simulink model "L1AdaptiveSystemModel"  (Simulink 7.3)
settings: Solver=ode45  StartTime=0.0  StopTime=30  RelTol=1e-3
InitFcn:
  | initL1AdaptiveSystemModel
StopFcn:
  | plotlab
values from neighbouring files (symbols this model uses):
  A = [0 1;0 0]    [initL1AdaptiveSystemModel.m]
  Am = A - b*km'    [initL1AdaptiveSystemModel.m]
  b = [0 ; d0]    [initL1AdaptiveSystemModel.m]
  c = [1 ; 1]    [initL1AdaptiveSystemModel.m]
  Cs_den = [1 25]    [initL1AdaptiveSystemModel.m]
  Cs_num = 25    [initL1AdaptiveSystemModel.m]
  Gamma = 100    [initL1AdaptiveSystemModel.m]
  kg = -(c'*(Am^-1)*b).^-1    [initL1AdaptiveSystemModel.m]
  km = [0.25 ; 0.707]    [initL1AdaptiveSystemModel.m]
  P = lyap(Am',Q)    [initL1AdaptiveSystemModel.m]
  theta = [0 -0.018 0.015 -0.062 0.0095 0.021]    [initL1AdaptiveSystemModel.m]
  theta2 = [4 -0.018 0.015 -0.062 0.0095 0.021]    [initL1AdaptiveSystemModel.m]
  ththat0 = zeros(6,1)    [initL1AdaptiveSystemModel.m]
  tNonlinChange = 10    [initL1AdaptiveSystemModel.m]
  tNonlinEnable = 0    [initL1AdaptiveSystemModel.m]
  x0 = zeros(2,1)    [initL1AdaptiveSystemModel.m]
  xhat0 = zeros(2,1)    [initL1AdaptiveSystemModel.m]
libraries: dspmtrx3 x4, simulink x3, Projection x1
settings Model: Creator=alp.marangoz  LastModifiedBy=Alp
settings OptimizationCC: ExpressionDepthLimit=128
settings DebuggingCC: StateNameClashWarn=none  StrictBusMsg=ErrorLevel1
settings CodeAppCC: CustomSymbolStrType=$N$R$M_T
settings GRTTargetCC: CombineOutputUpdateFcns=on

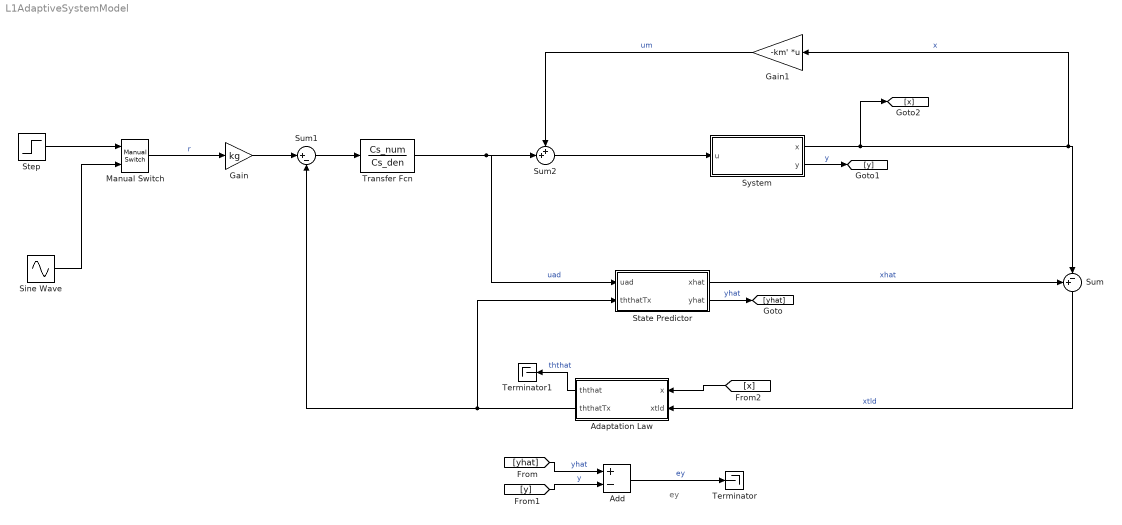
== system L1AdaptiveSystemModel ==
  note: ey
  Adaptation Law : Subsystem  TreatAsAtomicUnit=on
      settings: MinAlgLoopOccurrences=on
  Add : Sum  Inputs=+-  OutDataType=fixdt(1, 16)  OutScaling=2^-10
  Gain : Gain  Gain=kg  ParameterDataType=fixdt(1, 16)  ParameterScaling=2^0  OutDataType=fixdt(1, 16)  OutScaling=2^0
  Gain1 : Gain  Gain=-km'  Multiplication=Matrix(K*u)  ParameterDataType=fixdt(1, 16)  ParameterScaling=2^0  OutDataType=fixdt(1, 16)  OutScaling=2^0
  Manual Switch : simulink/Signal Routing/Manual Switch  SystemSampleTime=-1  sw=0  action=0  varsize=off
  Sine Wave : Sin  Amplitude=-2  Bias=0  Frequency=0.15  Phase=0  Samples=10  SampleTime=0  Offset=0
  State Predictor : Subsystem  TreatAsAtomicUnit=on
      settings: MinAlgLoopOccurrences=on
  Step : Step  SampleTime=0  VectorParams1D=off
  Sum : Sum  Inputs=+-|  OutDataType=fixdt(1, 16)  OutScaling=2^0
  Sum1 : Sum  Inputs=|+-  OutDataType=fixdt(1, 16)  OutScaling=2^0
  Sum2 : Sum  Inputs=++|  OutDataType=fixdt(1, 16)  OutScaling=2^0
  System : Subsystem  TreatAsAtomicUnit=on
      settings: MinAlgLoopOccurrences=on
  Terminator : Terminator
  Terminator1 : Terminator
  Transfer Fcn : TransferFcn  Numerator=Cs_num  Denominator=Cs_den
  wires:
  Sum/1 -> Adaptation Law/2(xtld)  "xtld"
  Manual Switch/1 -> Gain/1  "r"
  State Predictor/2(yhat) -> [yhat]  "yhat"
  System/2(y) -> [y]  "y"
  [yhat] -> Add/1  "yhat"
  [y] -> Add/2  "y"
  Add/1 -> Terminator/1  "ey"
  Step/1 -> Manual Switch/1
  Sine Wave/1 -> Manual Switch/2
  System/1(x) -> [x], Sum/2, Gain1/1  "x"
  Gain/1 -> Sum1/1
  State Predictor/1(xhat) -> Sum/1  "xhat"
  Sum1/1 -> Transfer Fcn/1
  Transfer Fcn/1 -> State Predictor/1(uad), Sum2/2  "uad"
  Adaptation Law/2(ththatTx) -> Sum1/2, State Predictor/2(ththatTx)
  Adaptation Law/1(ththat) -> Terminator1/1  "ththat"
  [x] -> Adaptation Law/1(x)
  Sum2/1 -> System/1(u)
  Gain1/1 -> Sum2/1  "um"

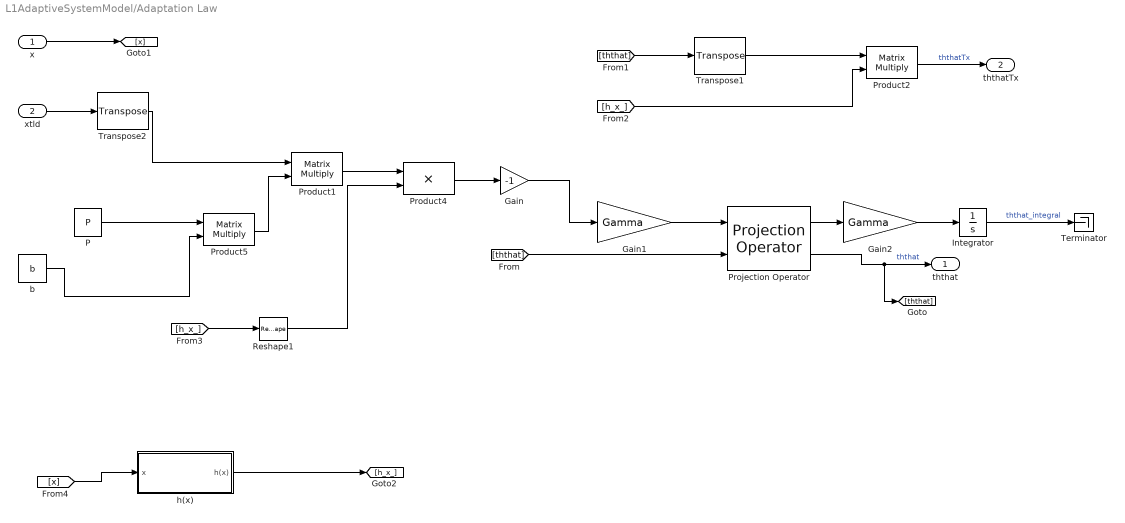
== system L1AdaptiveSystemModel/Adaptation Law ==
  x : Inport  OutDataType=fixdt(1, 16)  OutScaling=2^0
  xtld : Inport  Port=2  OutDataType=fixdt(1, 16)  OutScaling=2^0
  Gain : Gain  Gain=-1  ParameterDataType=fixdt(1, 16)  ParameterScaling=2^0  OutDataType=fixdt(1, 16)  OutScaling=2^0
  Gain1 : Gain  Gain=Gamma  ParameterDataType=fixdt(1, 16)  ParameterScaling=2^0  OutDataType=fixdt(1, 16)  OutScaling=2^0
  Gain2 : Gain  Gain=Gamma  ParameterDataType=fixdt(1, 16)  ParameterScaling=2^0  OutDataType=fixdt(1, 16)  OutScaling=2^0
  Integrator : Integrator  InitialCondition=ththat0
  P : Constant  Value=P  VectorParams1D=off  OutDataType=fixdt(1, 16)  OutScaling=2^0
  Product1 : Product  Multiplication=Matrix(*)  OutDataType=fixdt(1, 16)  OutScaling=2^0  RndMeth=Zero
  Product2 : Product  Multiplication=Matrix(*)  OutDataType=fixdt(1, 16)  OutScaling=2^0  RndMeth=Zero
  Product4 : Product  OutDataType=fixdt(1, 16)  OutScaling=2^0  RndMeth=Zero
  Product5 : Product  Multiplication=Matrix(*)  OutDataType=fixdt(1, 16)  OutScaling=2^0  RndMeth=Zero
  Projection Operator : Projection/Projection Operator  SystemSampleTime=-1  EpsilonTheta=.1  Prmax=1  Prcenter=0  Pr0=ththat0
  Reshape1 : Reshape  OutputDimensionality=Column vector (2-D)  OutputDimensions=[1]
  Terminator : Terminator
  Transpose1 : dspmtrx3/Transpose  SystemSampleTime=-1  Hermitian=off  overflowFlag=off
  Transpose2 : dspmtrx3/Transpose  SystemSampleTime=-1  Hermitian=off  overflowFlag=off
  b : Constant  Value=b  VectorParams1D=off  OutDataType=fixdt(1, 16)  OutScaling=2^0
  h(x) : Subsystem  TreatAsAtomicUnit=on
  ththat : Outport  OutDataType=fixdt(1, 16)  OutScaling=2^0
  ththatTx : Outport  Port=2  OutDataType=fixdt(1, 16)  OutScaling=2^0
  wires:
  P/1 -> Product5/1
  xtld/1 -> Transpose2/1
  Transpose2/1 -> Product1/1
  Product5/1 -> Product1/2
  b/1 -> Product5/2
  Gain/1 -> Gain1/1
  Gain1/1 -> Projection Operator/1
  Projection Operator/1 -> Gain2/1
  Gain2/1 -> Integrator/1
  Projection Operator/2 -> ththat/1, [ththat]  "ththat"
  Integrator/1 -> Terminator/1  "ththat_integral"
  Transpose1/1 -> Product2/1
  Product2/1 -> ththatTx/1  "ththatTx"
  [ththat] -> Transpose1/1
  [h_x_] -> Product2/2
  [ththat] -> Projection Operator/2
  x/1 -> [x]
  Product4/1 -> Gain/1
  [h_x_] -> Reshape1/1
  Reshape1/1 -> Product4/2
  Product1/1 -> Product4/1
  [x] -> h(x)/1(x)
  h(x)/1(h(x)) -> [h_x_]

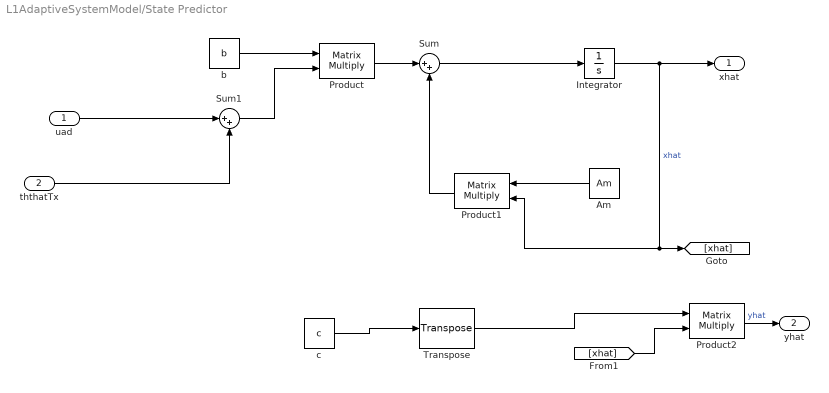
== system L1AdaptiveSystemModel/State Predictor ==
  uad : Inport  OutDataType=fixdt(1, 16)  OutScaling=2^0
  ththatTx : Inport  Port=2  OutDataType=fixdt(1, 16)  OutScaling=2^0
  Am : Constant  Value=Am  VectorParams1D=off  OutDataType=fixdt(1, 16)  OutScaling=2^0
  Integrator : Integrator  InitialCondition=xhat0
  Product : Product  Multiplication=Matrix(*)  OutDataType=fixdt(1, 16)  OutScaling=2^0  RndMeth=Zero
  Product1 : Product  Multiplication=Matrix(*)  OutDataType=fixdt(1, 16)  OutScaling=2^0  RndMeth=Zero
  Product2 : Product  Multiplication=Matrix(*)  OutDataType=fixdt(1, 16)  OutScaling=2^0  RndMeth=Zero
  Sum : Sum  Inputs=|++  OutDataType=fixdt(1, 16)  OutScaling=2^0
  Sum1 : Sum  Inputs=|++  OutDataType=fixdt(1, 16)  OutScaling=2^0
  Transpose : dspmtrx3/Transpose  SystemSampleTime=-1  Hermitian=off  overflowFlag=off
  b : Constant  Value=b  VectorParams1D=off  OutDataType=fixdt(1, 16)  OutScaling=2^0
  c : Constant  Value=c  VectorParams1D=off  OutDataType=fixdt(1, 16)  OutScaling=2^0
  xhat : Outport  OutDataType=fixdt(1, 16)  OutScaling=2^0
  yhat : Outport  Port=2  OutDataType=fixdt(1, 16)  OutScaling=2^0
  wires:
  c/1 -> Transpose/1
  Am/1 -> Product1/1
  Sum/1 -> Integrator/1
  Integrator/1 -> xhat/1, Product1/2, [xhat]  "xhat"
  Product1/1 -> Sum/2
  Product/1 -> Sum/1
  Transpose/1 -> Product2/1
  Product2/1 -> yhat/1  "yhat"
  b/1 -> Product/1
  Sum1/1 -> Product/2
  uad/1 -> Sum1/1
  [xhat] -> Product2/2
  ththatTx/1 -> Sum1/2

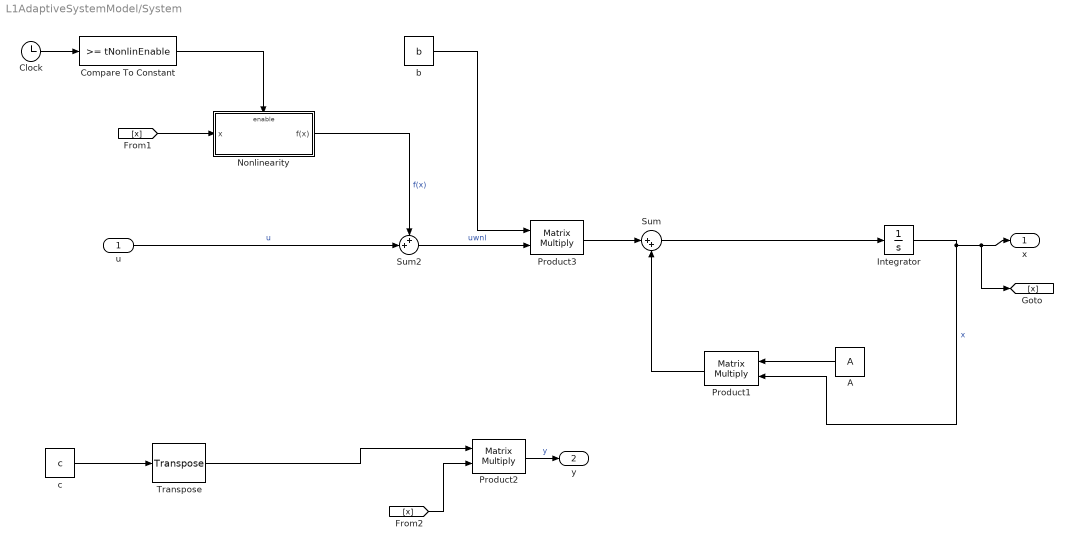
== system L1AdaptiveSystemModel/System ==
  u : Inport  OutDataType=fixdt(1, 16)  OutScaling=2^0
  A : Constant  Value=A  VectorParams1D=off  OutDataType=fixdt(1, 16)  OutScaling=2^0
  Clock : Clock
      settings: Decimation=10
  Compare To Constant : simulink/Logic and Bit Operations/Compare To Constant  SystemSampleTime=-1  relop=>=  const=tNonlinEnable  LogicOutDataTypeMode=uint8  ZeroCross=off
  Integrator : Integrator  InitialCondition=x0
  Nonlinearity : Subsystem  TreatAsAtomicUnit=on
  Product1 : Product  Multiplication=Matrix(*)  OutDataType=fixdt(1, 16)  OutScaling=2^0  RndMeth=Zero
  Product2 : Product  Multiplication=Matrix(*)  OutDataType=fixdt(1, 16)  OutScaling=2^0  RndMeth=Zero
  Product3 : Product  Multiplication=Matrix(*)  OutDataType=fixdt(1, 16)  OutScaling=2^0  RndMeth=Zero
  Sum : Sum  Inputs=|++  OutDataType=fixdt(1, 16)  OutScaling=2^0
  Sum2 : Sum  Inputs=++|  OutDataType=fixdt(1, 16)  OutScaling=2^0
  Transpose : dspmtrx3/Transpose  SystemSampleTime=-1  Hermitian=off  overflowFlag=off
  b : Constant  Value=b  VectorParams1D=off  OutDataType=fixdt(1, 16)  OutScaling=2^0
  c : Constant  Value=c  VectorParams1D=off  OutDataType=fixdt(1, 16)  OutScaling=2^0
  x : Outport  OutDataType=fixdt(1, 16)  OutScaling=2^0
  y : Outport  Port=2  OutDataType=fixdt(1, 16)  OutScaling=2^0
  wires:
  Product2/1 -> y/1  "y"
  Transpose/1 -> Product2/1
  Integrator/1 -> x/1, [x], Product1/2  "x"
  A/1 -> Product1/1
  c/1 -> Transpose/1
  [x] -> Nonlinearity/1(x)
  Clock/1 -> Compare To Constant/1
  Compare To Constant/1 -> Nonlinearity/Enable
  Nonlinearity/1(f(x)) -> Sum2/1  "f(x)"
  [x] -> Product2/2
  u/1 -> Sum2/2  "u"
  b/1 -> Product3/1
  Sum2/1 -> Product3/2  "uwnl"
  Product3/1 -> Sum/1
  Product1/1 -> Sum/2
  Sum/1 -> Integrator/1

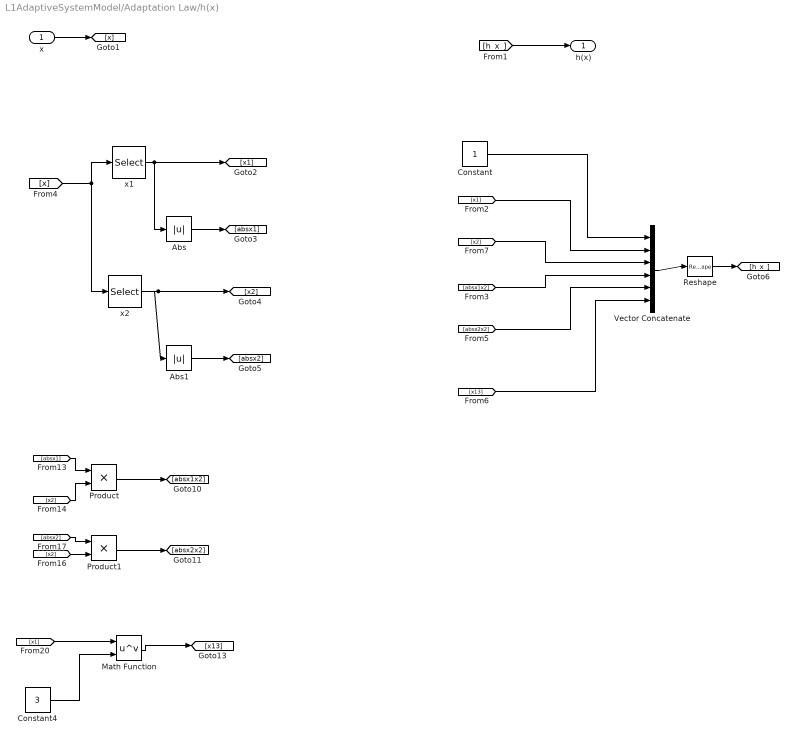
== system L1AdaptiveSystemModel/Adaptation Law/h(x) ==
  x : Inport  OutDataType=fixdt(1, 16)  OutScaling=2^0
  Abs : Abs  OutDataType=fixdt(1, 16)  OutScaling=2^0
  Abs1 : Abs  OutDataType=fixdt(1, 16)  OutScaling=2^0
  Constant : Constant  OutDataType=fixdt(1, 16)  OutScaling=2^0
  Constant4 : Constant  Value=3  VectorParams1D=off  OutDataType=fixdt(1, 16)  OutScaling=2^0
  Math Function : Math  Operator=pow  OutDataType=fixdt(1, 16)  OutScaling=2^0  SaturateOnIntegerOverflow=on
  Product : Product  OutDataType=fixdt(1, 16)  OutScaling=2^0  RndMeth=Zero
  Product1 : Product  OutDataType=fixdt(1, 16)  OutScaling=2^0  RndMeth=Zero
  Reshape : Reshape  OutputDimensionality=Column vector (2-D)
  Vector Concatenate : Concatenate  NumInputs=6  Mode=Vector
  x1 : Selector  InputPortWidth=2  IndexOptions=Index vector (dialog)  Indices=[1 ]  OutputSizes=1
  x2 : Selector  InputPortWidth=2  IndexOptions=Index vector (dialog)  Indices=2  OutputSizes=1
  h(x) : Outport  OutDataType=fixdt(1, 16)  OutScaling=2^0
  wires:
  [x] -> x2/1, x1/1
  x1/1 -> [x1], Abs/1
  Abs/1 -> [absx1]
  x2/1 -> [x2], Abs1/1
  Abs1/1 -> [absx2]
  x/1 -> [x]
  [h_x_] -> h(x)/1
  Vector Concatenate/1 -> Reshape/1
  [absx1] -> Product/1
  [x2] -> Product/2
  Product/1 -> [absx1x2]
  [absx2] -> Product1/1
  [x2] -> Product1/2
  Product1/1 -> [absx2x2]
  [x1] -> Math Function/1
  Constant4/1 -> Math Function/2
  Math Function/1 -> [x13]
  Reshape/1 -> [h_x_]
  Constant/1 -> Vector Concatenate/1
  [x1] -> Vector Concatenate/2
  [x2] -> Vector Concatenate/3
  [absx1x2] -> Vector Concatenate/4
  [absx2x2] -> Vector Concatenate/5
  [x13] -> Vector Concatenate/6

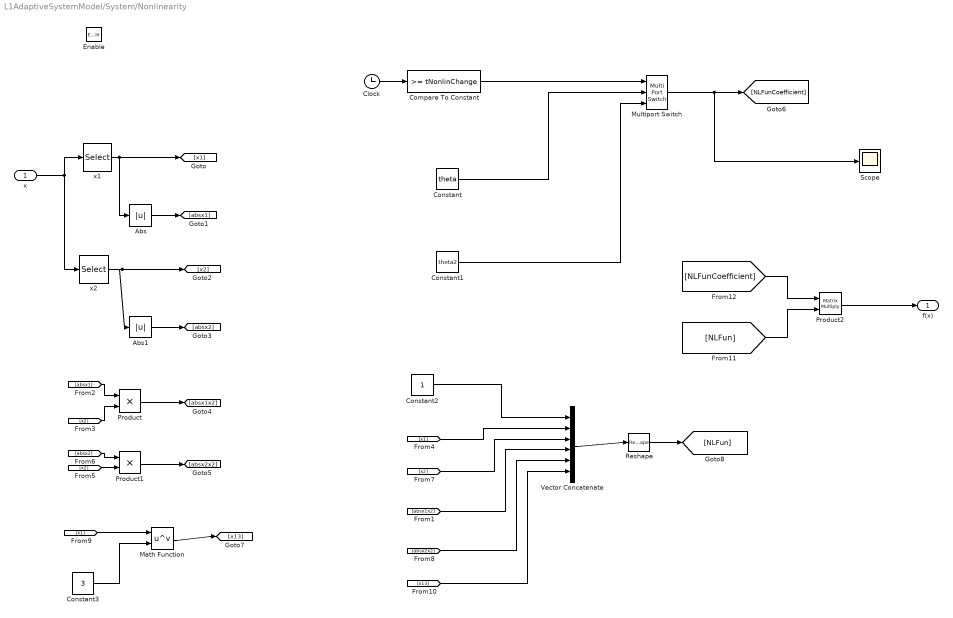
== system L1AdaptiveSystemModel/System/Nonlinearity ==
  x : Inport  OutDataType=fixdt(1, 16)  OutScaling=2^0
  Enable : EnablePort
  Abs : Abs  OutDataType=fixdt(1, 16)  OutScaling=2^0
  Abs1 : Abs  OutDataType=fixdt(1, 16)  OutScaling=2^0
  Clock : Clock
      settings: Decimation=10
  Compare To Constant : simulink/Logic and Bit Operations/Compare To Constant  SystemSampleTime=-1  relop=>=  const=tNonlinChange  LogicOutDataTypeMode=uint8  ZeroCross=off
  Constant : Constant  Value=theta  VectorParams1D=off  OutDataType=fixdt(1, 16)  OutScaling=2^0
  Constant1 : Constant  Value=theta2  VectorParams1D=off  OutDataType=fixdt(1, 16)  OutScaling=2^0
  Constant2 : Constant  VectorParams1D=off  OutDataType=fixdt(1, 16)  OutScaling=2^0
  Constant3 : Constant  Value=3  VectorParams1D=off  OutDataType=fixdt(1, 16)  OutScaling=2^0
  Math Function : Math  Operator=pow  OutDataType=fixdt(1, 16)  OutScaling=2^0  SaturateOnIntegerOverflow=on
  Multiport Switch : MultiPortSwitch  Inputs=2  zeroidx=on  OutDataType=fixdt(1, 16)  OutScaling=2^0
  Product : Product  OutDataType=fixdt(1, 16)  OutScaling=2^0  RndMeth=Zero
  Product1 : Product  OutDataType=fixdt(1, 16)  OutScaling=2^0  RndMeth=Zero
  Product2 : Product  Multiplication=Matrix(*)  OutDataType=fixdt(1, 16)  OutScaling=2^0  RndMeth=Zero
  Reshape : Reshape  OutputDimensionality=Column vector (2-D)
  Scope : Scope
  Vector Concatenate : Concatenate  NumInputs=6  Mode=Vector
  x1 : Selector  InputPortWidth=2  IndexOptions=Index vector (dialog)  Indices=[1 ]  OutputSizes=1
  x2 : Selector  InputPortWidth=2  IndexOptions=Index vector (dialog)  Indices=2  OutputSizes=1
  f(x) : Outport  OutDataType=fixdt(1, 16)  OutScaling=2^0
  wires:
  x/1 -> x2/1, x1/1
  x1/1 -> [x1], Abs/1
  Abs/1 -> [absx1]
  x2/1 -> [x2], Abs1/1
  Abs1/1 -> [absx2]
  [absx1] -> Product/1
  [x2] -> Product/2
  Product/1 -> [absx1x2]
  [absx2] -> Product1/1
  [x2] -> Product1/2
  Product1/1 -> [absx2x2]
  Clock/1 -> Compare To Constant/1
  Compare To Constant/1 -> Multiport Switch/1
  Constant/1 -> Multiport Switch/2
  Constant1/1 -> Multiport Switch/3
  Multiport Switch/1 -> [NLFunCoefficient], Scope/1
  [x1] -> Math Function/1
  Constant3/1 -> Math Function/2
  Math Function/1 -> [x13]
  Constant2/1 -> Vector Concatenate/1
  [x1] -> Vector Concatenate/2
  [x2] -> Vector Concatenate/3
  [absx1x2] -> Vector Concatenate/4
  [absx2x2] -> Vector Concatenate/5
  [x13] -> Vector Concatenate/6
  Vector Concatenate/1 -> Reshape/1
  [NLFunCoefficient] -> Product2/1
  [NLFun] -> Product2/2
  Product2/1 -> f(x)/1
  Reshape/1 -> [NLFun]
